simulink model "power_dcdrive_utku"  (R2015a)
settings: Solver=ode23tb  SolverMode=SingleTasking  StartTime=0.0  StopTime=2.5  RelTol=1e-4
InitFcn:
  | load power_dcdrive_init
libraries: powerlib x12
Description:
  | The 'Model  initialization function' defined in the
  | 
  | Model Properties loads the  initial states vector
  | 
  | 'xInitial' saved in the power_dcdrive_init.mat file.
  | 
  | 
  | 
  | To start in steady state with Speed = 120 rad/s
  | 
  | and Torque = 5 N.m/s, check 'Initial state' in
  | 
  | Simulation/Simulation parameters/Workspace I/O.
  | 
  | 
  | Copyright 2008-2015 The MathWorks, Inc.
settings Model: FPTRunName=Active  CovSFcnEnable=off  ExtModeTrigMode=oneshot  ExtModeArmWhenConnect=off  ExtModeAutoUpdateStatusClock=off  Creator=MathWorks  LastModifiedBy=UErdem
settings SolverCC: SolverResetMethod=Robust
settings DataIOCC: LimitDataPoints=off  SignalLoggingSaveFormat=ModelDataLogs  SaveOutput=off  SignalLogging=off  SaveTime=off  SignalLoggingName=sigsOut
settings OptimizationCC: BlockReduction=off  BooleanDataType=off  ExpressionDepthLimit=2147483647  InitFltsAndDblsToZero=on  EfficientMapNaN2IntZero=off
settings DebuggingCC: SaveWithParameterizedLinksMsg=none  UnderspecifiedInitializationDetection=Classic  MergeDetectMultiDrivingBlocksExec=none  CheckExecutionContextPreStartOutputMsg=on  CheckExecutionContextRuntimeOutputMsg=on  SignalResolutionControl=TryResolveAllWithWarning  MultiTaskDSMMsg=warning  MultiTaskCondExecSysMsg=none  FcnCallInpInsideContextMsg=UseLocalSettings  UnconnectedInputMsg=none  UnconnectedOutputMsg=none  StateNameClashWarn=warning
settings HardwareCC: TargetUnknown=on
settings GRTTargetCC: TargetFcnLib=ansi_tfl_tmw.mat  CombineOutputUpdateFcns=off  GRTInterface=on

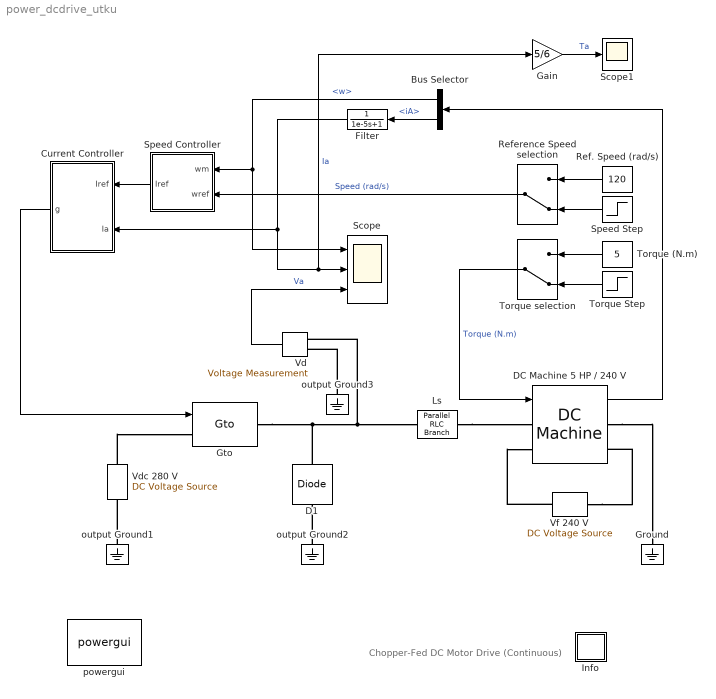
== system power_dcdrive_utku ==
  note: Chopper-Fed DC Motor Drive (Continuous)
  Bus Selector : BusSelector  OutputSignals=w,iA
  Current Controller : Subsystem  mask{h=2}
      mask prompts: h "Hysteresis band (A)"
      mask help: Hysteresis Current Controller
      mask Display: plot(0,0,100,100,[45,45],[35,65],[55,55],[35,65],[45,65],[65,65],[35,55],[35,35])
  D1 : powerlib/Power Electronics/Diode  Ron=0.05  Lon=0  Vf=0.7  IC=0  UseSnubber=off  Rs=Inf  Cs=0.1e-6  Measurements=off
  DC Machine 5 HP / 240 V : powerlib/Machines/DC Machine  PresetModel=No  MechanicalLoad=Torque TL  FieldType=Wound  ShowDetailedParameters=on  MeasurementBus=on  RLa="[ 0.5  0.01]"  RLf="[ 240  120]"  Laf=1.23  MachineConstant=Torque constant (N.m/A)  Ke=1.8  Kt=1.8  J=0.05  Bm=0.02  Tf=0  w0=0.1  Ifinit=0  TsPowergui=0  TsBlock=-1
  Filter : TransferFcn  Numerator=1  Denominator=[1e-5 1]
      mask Display: disp('Filter')
  Gain : Gain  Gain=5/6
  Ground : powerlib/Elements/Ground  LConnTagsString=a
  Gto : powerlib/Power Electronics/Gto  Ron=0.05  Lon=0  Vf=1  Tf=1e-6  Tt=1e-6  IC=0  Rs=1e4  Cs=inf  Measurements=off
      settings: AttributesFormatString=\n
  Info : Subsystem
      settings: OpenFcn=showdemo(bdroot(gcb))
      mask Display: disp('?')
  Ls : powerlib/Elements/Parallel RLC Branch  LConnTagsString=a  RConnTagsString=__new0  BranchType=L  Resistance=[]  Inductance=10e-03  SetiL0=off  InitialCurrent=0  Capacitance=[]  Setx0=off  InitialVoltage=0  Measurements=None
  Ref. Speed (rad/s) : Constant  Value=120
  Reference Speed selection : ManualSwitch  CurrentSetting=0
  Scope : Scope  NumInputPorts=3
      settings: TimeRange=2.5  YMin=0~0~-100  YMax=150~40~300
  Scope1 : Scope
  Speed Controller : Subsystem  mask(PI controller){Kp=1.6, Ki=16, Ilim=30}
      mask prompts: Kp "Proportional gain (Kp)"; Ki "Integral gain (Ki)"; Ilim "Current limit (A)"
      mask help: Proportional-Integral Speed Controller
      mask Display: plot(0,0,100,100,[35,35,65],[70,30,30],[35,65],[45,60])
  Speed Step : Step  Time=0.4  Before=120  After=160  SampleTime=0
  Torque selection : ManualSwitch  CurrentSetting=0
  Torque (N.m) : Constant  Value=5
  Torque Step : Step  Time=1.2  Before=5  After=25  SampleTime=0
  Vd : powerlib/Measurements/Voltage Measurement  Tag=PoWeRsYsTeMmEaSuReMeNt  PhasorSimulation=off  OutputType=Magnitude  PSBequivalent=0
  "Vdc 280 V " : powerlib/Electrical Sources/DC Voltage Source  Description=source block  Amplitude=280  Measurements=None
      settings: AttributesFormatString=\n
  Vf 240 V : powerlib/Electrical Sources/DC Voltage Source  Description=source block  Amplitude=240  Measurements=None
      settings: AttributesFormatString=\n
  output Ground1 : powerlib/Elements/Ground  LConnTagsString=a
  output Ground2 : powerlib/Elements/Ground  LConnTagsString=a
  output Ground3 : powerlib/Elements/Ground  LConnTagsString=a
  powergui : powerlib/powergui  SimulationMode=Continuous  SolverType=Tustin  SampleTime=0  frequency=60  SPID=on  DisableSnubberDevices=on  DisableRonSwitches=off  DisableVfSwitches=off  SwTol=0  DisplayEquations=off  Interpol=off  methode=off  Ts=0  FunctionMessages=off  echomessages=off  HookPort=off  EnableUseOfTLC=off  x0status=blocks  frequencyindice=0  Pbase=100e6  ErrMax=1e-4  Iterations=50  UnitsV=kV  UnitsW=MW  buscounter=0  RestoreLinks=warning  ResistiveCurrentMeasurement=off  Frange=[0:2:500]  Ylog=off  Xlog=on  ShowGrid=off  save=off  variable=ZData  structure=0  ZoomFFT=on  StartTime=0.0  cycles=1  DisplayStyle=1  fundamental=60  FreqAxis=off  MaxFrequency=1000  frequencyindicesteady=1  RmsSteady=1  display=off
  wires:
  Speed Controller/1(Iref) -> Current Controller/1(Iref)
  Filter/1 -> Gain/1, Scope/2, Current Controller/2(Ia)  "Ia"
  Bus Selector/1 -> Scope/1, Speed Controller/1(wm)  "<w>"
  Bus Selector/2 -> Filter/1  "<iA>"
  Current Controller/1(g) -> Gto/1
  Vd/1 -> Scope/3  "Va"
  DC Machine 5 HP / 240 V/1 -> Bus Selector/1
  Torque (N.m)/1 -> Torque selection/1
  Torque Step/1 -> Torque selection/2
  Torque selection/1 -> DC Machine 5 HP / 240 V/1  "Torque (N.m)"
  Reference Speed selection/1 -> Speed Controller/2(wref)  "Speed (rad/s)"
  Ref. Speed (rad/s)/1 -> Reference Speed selection/1
  Speed Step/1 -> Reference Speed selection/2
  Gain/1 -> Scope1/1  "Ta"
  connections:
  output Ground2/LConn1 -- D1/LConn1
  Gto/RConn1 -- Ls/LConn1 -- Vd/LConn1 -- D1/RConn1
  "Vdc 280 V "/RConn1 -- Gto/LConn1
  output Ground1/LConn1 -- "Vdc 280 V "/LConn1
  Ls/RConn1 -- DC Machine 5 HP / 240 V/LConn1
  output Ground3/LConn1 -- Vd/LConn2
  DC Machine 5 HP / 240 V/RConn1 -- Ground/LConn1
  Vf 240 V/LConn1 -- DC Machine 5 HP / 240 V/RConn2
  Vf 240 V/RConn1 -- DC Machine 5 HP / 240 V/LConn2

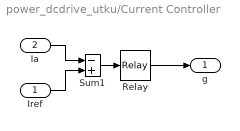
== system power_dcdrive_utku/Current Controller ==
  Iref : Inport
  Ia : Inport  Port=2
  Relay : Relay  OnSwitchValue=h/2  OffSwitchValue=-h/2
  Sum1 : Sum  Inputs=-+  SaturateOnIntegerOverflow=on  InputSameDT=on  OutDataTypeStr=Inherit: Same as first input
  g : Outport  InitialOutput=0
  wires:
  Sum1/1 -> Relay/1
  Relay/1 -> g/1
  Ia/1 -> Sum1/1
  Iref/1 -> Sum1/2

== system power_dcdrive_utku/Info ==

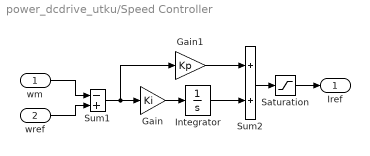
== system power_dcdrive_utku/Speed Controller ==
  wm : Inport
  wref : Inport  Port=2
  Gain : Gain  Gain=Ki  SaturateOnIntegerOverflow=on  OutDataTypeStr=Inherit: Same as input  ParamDataTypeStr=Inherit: Same as input
  Gain1 : Gain  Gain=Kp  SaturateOnIntegerOverflow=on  OutDataTypeStr=Inherit: Same as input  ParamDataTypeStr=Inherit: Same as input
  Integrator : Integrator  LimitOutput=on  UpperSaturationLimit=Ilim  LowerSaturationLimit=-Ilim
  Saturation : Saturate  UpperLimit=Ilim  LowerLimit=-Ilim
  Sum1 : Sum  Inputs=-+  SaturateOnIntegerOverflow=on  InputSameDT=on  OutDataTypeStr=Inherit: Same as first input
  Sum2 : Sum  SaturateOnIntegerOverflow=on  InputSameDT=on  OutDataTypeStr=Inherit: Same as first input
  Iref : Outport  InitialOutput=0
  wires:
  Saturation/1 -> Iref/1
  Sum2/1 -> Saturation/1
  Integrator/1 -> Sum2/2
  wref/1 -> Sum1/2
  wm/1 -> Sum1/1
  Sum1/1 -> Gain1/1, Gain/1
  Gain/1 -> Integrator/1
  Gain1/1 -> Sum2/1
